simulink model "canon"  (Simulink 10.0)
settings: Solver=ode45  StartTime=0.0  StopTime=10.0  RelTol=1e-3  EnableMultiTasking=on
undefined symbols (not defined in the file): g, teta, vox, voy, xo, yo
settings Model: Creator=unknown  LastModifiedBy=bhisma
settings DataIOCC: LimitDataPoints=on  SignalLoggingSaveFormat=ModelDataLogs
settings OptimizationCC: InitFltsAndDblsToZero=on
settings DebuggingCC: SaveWithParameterizedLinksMsg=none  SignalResolutionControl=TryResolveAllWithWarning  SolverPrmCheckMsg=warning  MultiTaskDSMMsg=warning  MultiTaskCondExecSysMsg=none
settings SFSimCC: SimUseLocalCustomCode=on  SimParseCustomCode=off  CustomCodeUndefinedFunction=FilterOut
settings RTWCC: RTWUseLocalCustomCode=on
settings GRTTargetCC: TargetFcnLib=ansi_tfl_tmw.mat

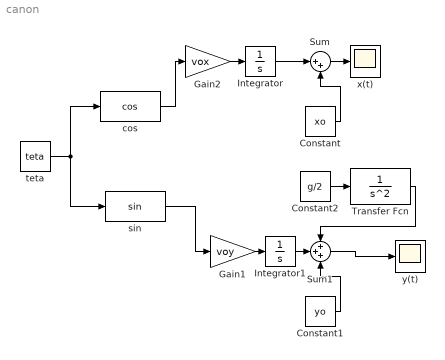
== system canon ==
  Constant : Constant  Value=xo
  Constant1 : Constant  Value=yo
  Constant2 : Constant  Value=g/2
  Gain1 : Gain  Gain=voy
  Gain2 : Gain  Gain=vox
  Integrator : Integrator
  Integrator1 : Integrator
  Sum : Sum  Inputs=|++
  Sum1 : Sum  Inputs=+++
  Transfer Fcn : TransferFcn  Denominator=[1 0 0]
  cos : MATLABFcn  MATLABFcn=cos
  sin : MATLABFcn
  teta : Constant  Value=teta
  x(t) : Scope
  y(t) : Scope
  wires:
  Integrator/1 -> Sum/1
  Sum/1 -> x(t)/1
  Constant/1 -> Sum/2
  Constant1/1 -> Sum1/3
  Sum1/1 -> y(t)/1
  sin/1 -> Gain1/1
  teta/1 -> cos/1, sin/1
  Gain1/1 -> Integrator1/1
  Integrator1/1 -> Sum1/2
  Constant2/1 -> Transfer Fcn/1
  Transfer Fcn/1 -> Sum1/1
  cos/1 -> Gain2/1
  Gain2/1 -> Integrator/1
